simulink model "VPP"  (R2020b)
settings: Solver=ode45  StartTime=0.0  StopTime=24  RelTol=1e-3  EnableMultiTasking=on
settings Model: Creator=persian  LastModifiedBy=Javad
settings DataIOCC: LimitDataPoints=on  SaveFormat=Array  ReturnWorkspaceOutputs=off
settings OptimizationCC: LifeSpan=inf
settings DebuggingCC: SolverPrmCheckMsg=warning  InitInArrayFormatMsg=none  SFUnexpectedBacktrackingDiag=warning  SFNoUnconditionalDefaultTransitionDiag=warning  SFExecutionAtInitializationDiag=none  ArithmeticOperatorsInVariantConditions=warning
settings HardwareCC: ProdBitPerPointer=32  ProdBitPerSizeT=32  ProdBitPerPtrDiffT=32  ProdLargestAtomicFloat=None  ProdIntDivRoundTo=Undefined  ProdEndianess=Unspecified  ProdWordSize=32  ProdHWDeviceType=32-bit Generic
settings ModelReferenceCC: PropagateSignalLabelsOutOfModel=off
settings SFSimCC: SimUseLocalCustomCode=off  CustomCodeUndefinedFunction=UseInterfaceOnly
settings RTWCC: RTWUseLocalCustomCode=off
settings CodeAppCC: StateflowObjectComments=on
settings GRTTargetCC: TargetLangStandard=C89/C90 (ANSI)
settings ConfigComp: CovMetricSettings=dw  CovSaveCumulativeToWorkspaceVar=on  CovSaveSingleToWorkspaceVar=on  CovExternalEMLEnable=off  CovSFcnEnable=off

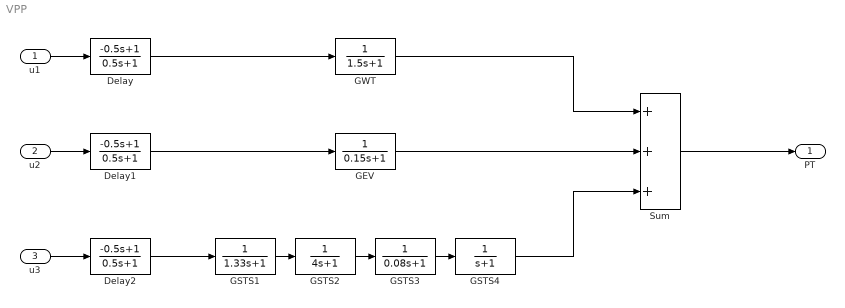
== system VPP ==
  u1 : Inport
  u2 : Inport  Port=2
  u3 : Inport  Port=3
  Delay : TransferFcn  Numerator=[-0.5 1]  Denominator=[0.5 1]
  Delay1 : TransferFcn  Numerator=[-0.5 1]  Denominator=[0.5 1]
  Delay2 : TransferFcn  Numerator=[-0.5 1]  Denominator=[0.5 1]
  GEV : TransferFcn  Denominator=[0.15 1]
  GSTS1 : TransferFcn  Denominator=[1.33 1]
  GSTS2 : TransferFcn  Denominator=[4 1]
  GSTS3 : TransferFcn  Denominator=[0.08 1]
  GSTS4 : TransferFcn  Denominator=[1 1]
  GWT : TransferFcn  Denominator=[1.5 1]
  Sum : Sum  Inputs=+++
  PT : Outport
  wires:
  GSTS3/1 -> GSTS4/1
  GSTS2/1 -> GSTS3/1
  GSTS1/1 -> GSTS2/1
  u1/1 -> Delay/1
  Delay/1 -> GWT/1
  GSTS4/1 -> Sum/3
  GEV/1 -> Sum/2
  GWT/1 -> Sum/1
  Delay1/1 -> GEV/1
  u2/1 -> Delay1/1
  Delay2/1 -> GSTS1/1
  u3/1 -> Delay2/1
  Sum/1 -> PT/1
